simulink model "svpwmadria"  (R2013a)
settings: Solver=ode45  StartTime=0.0  StopTime=10.0  RelTol=1e-3
undefined symbols (not defined in the file): T
libraries: simulink x1
settings Model: Creator=ajunyent  LastModifiedBy=ajunyent

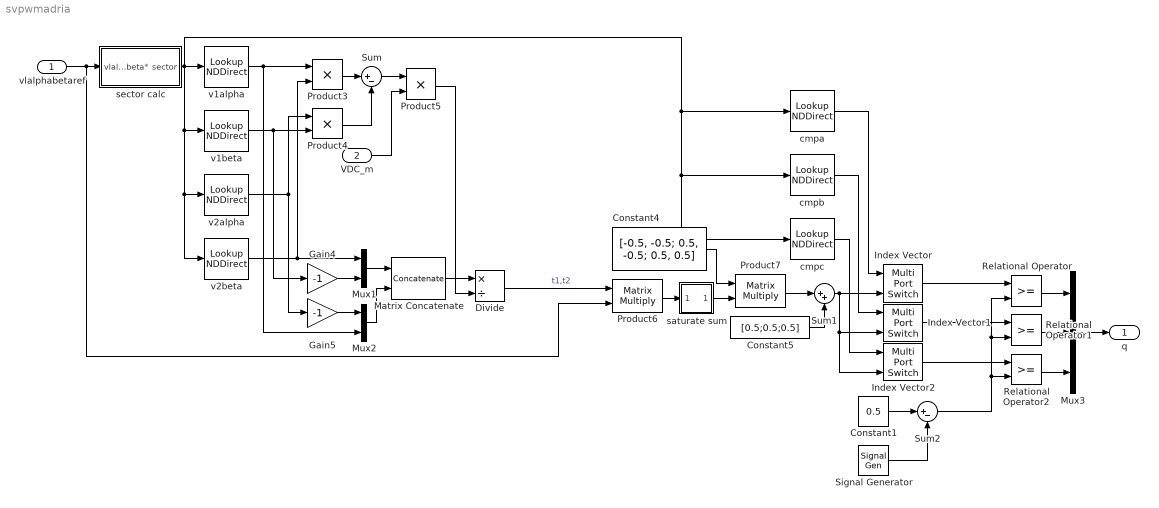
== system svpwmadria ==
  vlalphabetaref : Inport  PortDimensions=2
  VDC_m : Inport  Port=2
  Constant1 : Constant  Value=0.5
  Constant4 : Constant  Value=[-0.5, -0.5; 0.5, -0.5; 0.5, 0.5]  SampleTime=T
  Constant5 : Constant  Value=[0.5;0.5;0.5]  SampleTime=T
  Divide : Product  Inputs=*/
  Gain4 : Gain  Gain=-1
  Gain5 : Gain  Gain=-1
  Index Vector : MultiPortSwitch  DataPortOrder=Zero-based contiguous  Inputs=1  zeroidx=on
  Index Vector1 : MultiPortSwitch  DataPortOrder=Zero-based contiguous  Inputs=1  zeroidx=on
  Index Vector2 : MultiPortSwitch  DataPortOrder=Zero-based contiguous  Inputs=1  zeroidx=on
  Matrix Concatenate : Concatenate  Mode=Multidimensional array  ConcatenateDimension=2
  Mux1 : Mux  Inputs=2
  Mux2 : Mux  Inputs=2
  Mux3 : Mux  Inputs=3
  Product3 : Product  RndMeth=Zero
  Product4 : Product  RndMeth=Zero
  Product5 : Product  RndMeth=Zero
  Product6 : Product  Multiplication=Matrix(*)  RndMeth=Zero
  Product7 : Product  Multiplication=Matrix(*)  RndMeth=Zero
  Relational Operator : RelationalOperator  OutDataTypeStr=boolean
  Relational Operator1 : RelationalOperator  OutDataTypeStr=boolean
  Relational Operator2 : RelationalOperator  OutDataTypeStr=boolean
  Signal Generator : SignalGenerator  WaveForm=sawtooth  Amplitude=0.5  Frequency=1e3
  Sum : Sum  Inputs=|+-
  Sum1 : Sum  Inputs=|++
  Sum2 : Sum  Inputs=|+-
  cmpa : LookupNDDirect  NumberOfTableDimensions=1  Table=[2,1,0,0,1,2]
  cmpb : LookupNDDirect  NumberOfTableDimensions=1  Table=[1,2,2,1,0,0]
  cmpc : LookupNDDirect  NumberOfTableDimensions=1  Table=[0,0,1,2,2,1]
  saturate sum : Subsystem
  sector calc : Subsystem
  v1alpha : LookupNDDirect  NumberOfTableDimensions=1  Table=[1/3,1/3,-2/3,-2/3,1/3,1/3]
  v1beta : LookupNDDirect  NumberOfTableDimensions=1  Table=[-sqrt(3)/3,-sqrt(3)/3,0,0,sqrt(3)/3,sqrt(3)/3]
  v2alpha : LookupNDDirect  NumberOfTableDimensions=1  Table=[2/3,-1/3,-1/3,-1/3,-1/3,2/3]
  v2beta : LookupNDDirect  NumberOfTableDimensions=1  Table=[0,-sqrt(3)/3,-sqrt(3)/3,sqrt(3)/3,sqrt(3)/3,0]
  q : Outport
  wires:
  sector calc/1(sector) -> v1alpha/1, v1beta/1, v2alpha/1, v2beta/1, cmpa/1, cmpb/1, cmpc/1
  v1alpha/1 -> Product3/1, Mux2/2
  v2alpha/1 -> Product4/1, Gain5/1
  v1beta/1 -> Product4/2, Gain4/1
  v2beta/1 -> Product3/2, Mux1/1
  Product3/1 -> Sum/1
  Product4/1 -> Sum/2
  Sum/1 -> Product5/1
  Gain4/1 -> Mux1/2
  Gain5/1 -> Mux2/1
  Mux1/1 -> Matrix Concatenate/1
  Mux2/1 -> Matrix Concatenate/2
  Matrix Concatenate/1 -> Divide/1
  Product5/1 -> Divide/2
  Divide/1 -> Product6/1  "t1,t2"
  Product6/1 -> saturate sum/1(in)
  saturate sum/1(out) -> Product7/2
  Constant4/1 -> Product7/1
  Product7/1 -> Sum1/1
  Constant5/1 -> Sum1/2
  Sum1/1 -> Index Vector/2, Index Vector2/2, Index Vector1/2
  cmpc/1 -> Index Vector2/1
  cmpb/1 -> Index Vector1/1
  cmpa/1 -> Index Vector/1
  Index Vector/1 -> Relational Operator/1
  Index Vector1/1 -> Relational Operator1/1
  Index Vector2/1 -> Relational Operator2/1
  Sum2/1 -> Relational Operator/2, Relational Operator1/2, Relational Operator2/2
  Relational Operator/1 -> Mux3/1
  Relational Operator1/1 -> Mux3/2
  Relational Operator2/1 -> Mux3/3
  vlalphabetaref/1 -> Product6/2, sector calc/1(vlalphabeta*)
  VDC_m/1 -> Product5/2
  Mux3/1 -> q/1
  Constant1/1 -> Sum2/1
  Signal Generator/1 -> Sum2/2

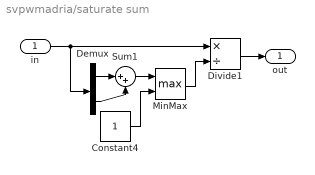
== system svpwmadria/saturate sum ==
  in : Inport
  Constant4 : Constant  SampleTime=T
  Demux : Demux  Outputs=2
  Divide1 : Product  Inputs=*/
  MinMax : MinMax  Function=max  Inputs=2
  Sum1 : Sum  Inputs=|++
  out : Outport
  wires:
  in/1 -> Divide1/1, Demux/1
  Demux/1 -> Sum1/1
  Sum1/1 -> MinMax/1
  Constant4/1 -> MinMax/2
  MinMax/1 -> Divide1/2
  Divide1/1 -> out/1
  Demux/2 -> Sum1/2

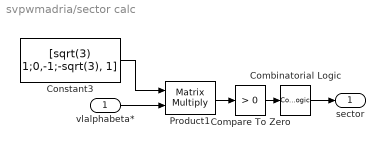
== system svpwmadria/sector calc ==
  vlalphabeta* : Inport
  Combinatorial Logic : CombinatorialLogic  TruthTable=[3;3;1;2;5;4;0;0]  SampleTime=T
  Compare To Zero : simulink/Logic and Bit Operations/Compare To Zero  relop=>  OutDataTypeStr=boolean  ZeroCross=off
  Constant3 : Constant  Value=[sqrt(3) 1;0,-1;-sqrt(3), 1]  SampleTime=T
  Product1 : Product  Multiplication=Matrix(*)  RndMeth=Zero
  sector : Outport
  wires:
  Constant3/1 -> Product1/1
  Product1/1 -> Compare To Zero/1
  Compare To Zero/1 -> Combinatorial Logic/1
  Combinatorial Logic/1 -> sector/1
  vlalphabeta*/1 -> Product1/2
